simulink library "SendToInputDevice"  (R2016b)
settings: Solver=VariableStepAuto  StartTime=0.0  StopTime=10.0  RelTol=1e-3
settings Model: Creator=Nathan  LastModifiedBy=march

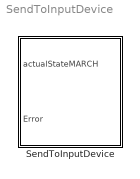
== system SendToInputDevice ==
  SendToInputDevice : Subsystem

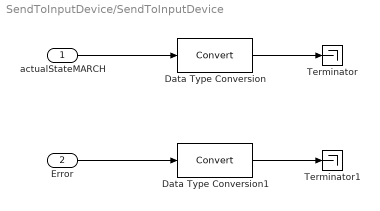
== system SendToInputDevice/SendToInputDevice ==
  actualStateMARCH : Inport
  Error : Inport  Port=2
  Data Type Conversion : DataTypeConversion
  Data Type Conversion1 : DataTypeConversion
  Terminator : Terminator
  Terminator1 : Terminator
  wires:
  Data Type Conversion1/1 -> Terminator1/1
  Data Type Conversion/1 -> Terminator/1
  Error/1 -> Data Type Conversion1/1
  actualStateMARCH/1 -> Data Type Conversion/1
